simulink subsystem "BatteryHVBasicRefSub"  (R2020a)
settings: Solver=VariableStepAuto  StartTime=0.0  StopTime=10.0  RelTol=1e-3
undefined symbols (not defined in the file or in its folder): battery
libraries: fl_lib x9, nesl_utility x4
settings Model: Creator=isaacito  LastModifiedBy=isaacito

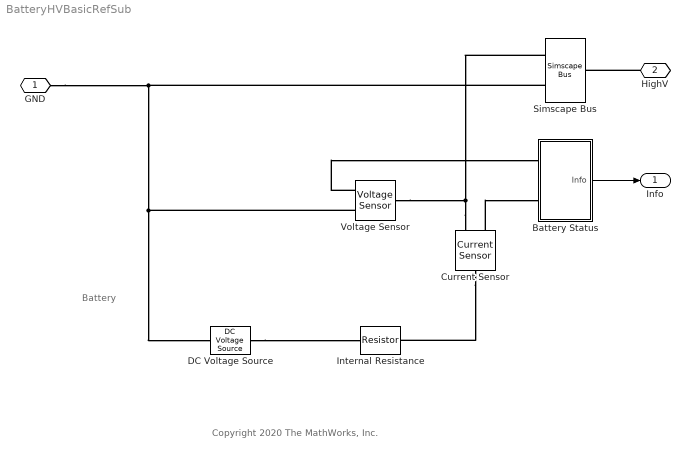
== system BatteryHVBasicRefSub ==
  note: Battery
  note: Copyright 2020 The MathWorks, Inc.
  Battery Status : Subsystem
  Current Sensor : fl_lib/Electrical/Electrical Sensors/Current Sensor
  DC Voltage Source : fl_lib/Electrical/Electrical Sources/DC Voltage Source  v0=battery.voltage_V V
      settings: AttributesFormatString=%<v0> %<v0_unit>
  Internal Resistance : fl_lib/Electrical/Electrical Elements/Resistor  R=battery.internal_R_Ohm Ohm  i_specify=off  i_priority=High  i=0 A  i_nominal_specify=off  i_nominal_unit=A  i_nominal_value=1  v_specify=off  v_priority=High  v=0 V  v_nominal_specify=off  v_nominal_unit=V  v_nominal_value=1
      settings: AttributesFormatString=%<R> %<R_unit>
  Simscape Bus : SimscapeBus  HierarchyStrings=plus;minus
  Voltage Sensor : fl_lib/Electrical/Electrical Sensors/Voltage Sensor
  GND : PMIOPort  Side=Left
  HighV : PMIOPort  Port=2  Side=Right
  Info : Outport
  wires:
  Battery Status/1(Info) -> Info/1
  connections:
  Voltage Sensor/RConn2 -- Simscape Bus/LConn2 -- GND/RConn1 -- DC Voltage Source/RConn1
  Current Sensor/RConn2 -- Voltage Sensor/LConn1 -- Simscape Bus/LConn1
  Current Sensor/RConn1 -- Battery Status/LConn2
  Current Sensor/LConn1 -- Internal Resistance/RConn1
  DC Voltage Source/LConn1 -- Internal Resistance/LConn1
  Voltage Sensor/RConn1 -- Battery Status/LConn1
  HighV/RConn1 -- Simscape Bus/RConn1

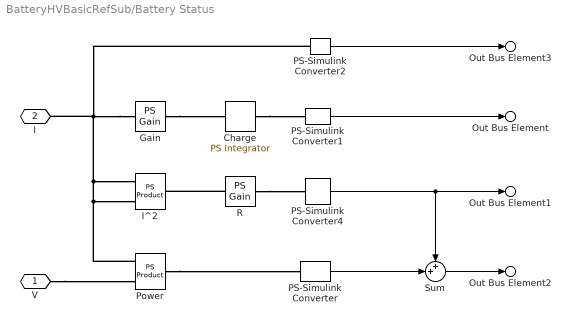
== system BatteryHVBasicRefSub/Battery Status ==
  Charge : fl_lib/Physical Signals/Linear Operators/PS Integrator  x0=50 A*hr
      settings: SourceProductBaseCode=SS
  Gain : fl_lib/Physical Signals/Functions/PS Gain  gain=-1
      settings: AttributesFormatString=%<gain>
  I^2 : fl_lib/Physical Signals/Functions/PS Product
  PS-Simulink Converter : nesl_utility/PS-Simulink Converter  PhysicalDomain=network_engine_domain  SubClassName=ps_output  LeftPortType=input  RightPortType=output  PseudoPeriodic=off  Frequencies=[]  Unit=kW  AffineConversion=off
  PS-Simulink Converter1 : nesl_utility/PS-Simulink Converter  PhysicalDomain=network_engine_domain  SubClassName=ps_output  LeftPortType=input  RightPortType=output  PseudoPeriodic=off  Frequencies=[]  Unit=A*hr  AffineConversion=off
  PS-Simulink Converter2 : nesl_utility/PS-Simulink Converter  PhysicalDomain=network_engine_domain  SubClassName=ps_output  LeftPortType=input  RightPortType=output  PseudoPeriodic=off  Frequencies=[]  Unit=A  AffineConversion=off
  PS-Simulink Converter4 : nesl_utility/PS-Simulink Converter  PhysicalDomain=network_engine_domain  SubClassName=ps_output  LeftPortType=input  RightPortType=output  PseudoPeriodic=off  Frequencies=[]  Unit=kW  AffineConversion=off
  Power : fl_lib/Physical Signals/Functions/PS Product
  R : fl_lib/Physical Signals/Functions/PS Gain  gain=battery.internal_R_Ohm Ohm
      settings: AttributesFormatString=%<gain> %<gain_unit>
  Sum : Sum  Inputs=++|
  V : PMIOPort  Side=Left
  I : PMIOPort  Port=2  Side=Left
  Out Bus Element : Outport  PortName=Info  Element=Charge
      settings: AttributesFormatString=%<Unit>
  Out Bus Element1 : Outport  PortName=Info  Element=PowerLoss
      settings: AttributesFormatString=%<Unit>
  Out Bus Element2 : Outport  PortName=Info  Element=Power
      settings: AttributesFormatString=%<Unit>
  Out Bus Element3 : Outport  PortName=Info  Element=Current
      settings: AttributesFormatString=%<Unit>
  wires:
  PS-Simulink Converter2/1 -> Out Bus Element3/1
  PS-Simulink Converter/1 -> Sum/2
  Sum/1 -> Out Bus Element2/1
  PS-Simulink Converter1/1 -> Out Bus Element/1
  PS-Simulink Converter4/1 -> Sum/1, Out Bus Element1/1
  connections:
  Gain/RConn1 -- Charge/LConn1
  Charge/RConn1 -- PS-Simulink Converter1/LConn1
  Power/RConn1 -- PS-Simulink Converter/LConn1
  V/RConn1 -- Power/LConn1
  Gain/LConn1 -- I^2/LConn2 -- I^2/LConn1 -- Power/LConn2 -- PS-Simulink Converter2/LConn1 -- I/RConn1
  R/LConn1 -- I^2/RConn1
  R/RConn1 -- PS-Simulink Converter4/LConn1
